simulink model "dip_student_sim_simulink_r2017b"  (R2017b)
settings: Solver=ode45  StartTime=0.0  StopTime=10  FixedStep=0.01  MaxStep=0.05  RelTol=1e-3  EnableMultiTasking=on
values from neighbouring files (symbols this model uses):
  x0 = [xR; 0; phi1R; 0; phi2R; 0]    [dip_student_sim_ini.m]
settings Model: Creator=ut  LastModifiedBy=15043
settings DataIOCC: LimitDataPoints=on  SaveFormat=Array  SignalLoggingSaveFormat=ModelDataLogs
settings OptimizationCC: ExpressionDepthLimit=2147483647  InitFltsAndDblsToZero=on  LifeSpan=inf
settings DebuggingCC: SaveWithParameterizedLinksMsg=none  UnderspecifiedInitializationDetection=Classic  MergeDetectMultiDrivingBlocksExec=none  SignalResolutionControl=TryResolveAllWithWarning  SolverPrmCheckMsg=warning  MultiTaskDSMMsg=warning  MultiTaskCondExecSysMsg=none  FcnCallInpInsideContextMsg=warning  StateNameClashWarn=warning  SFUnexpectedBacktrackingDiag=warning  SFNoUnconditionalDefaultTransitionDiag=warning  SFExecutionAtInitializationDiag=none
settings HardwareCC: ProdBitPerPointer=32  ProdBitPerSizeT=32  ProdBitPerPtrDiffT=32  ProdLargestAtomicFloat=None  ProdIntDivRoundTo=Undefined  ProdEndianess=Unspecified  ProdWordSize=32  ProdHWDeviceType=32-bit Generic
settings ModelReferenceCC: PropagateSignalLabelsOutOfModel=off
settings CodeAppCC: StateflowObjectComments=on
settings GRTTargetCC: TargetFcnLib=ansi_tfl_tmw.mat  TargetLangStandard=C89/C90 (ANSI)  CombineOutputUpdateFcns=off  GRTInterface=on
settings ConfigComp: CovMetricSettings=dw  CovSaveCumulativeToWorkspaceVar=on  CovSaveSingleToWorkspaceVar=on  CovExternalEMLEnable=off

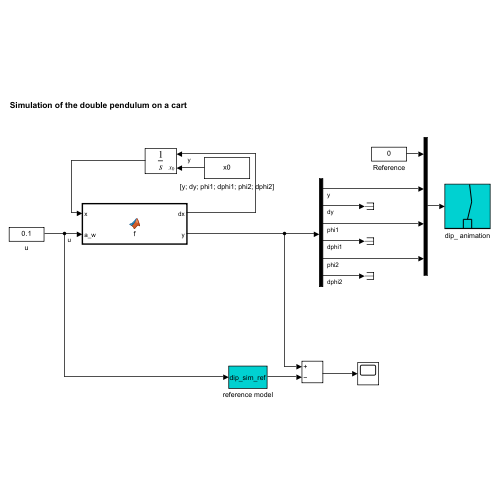
[thumbnail: Simulink's stored preview of the top-level diagram]
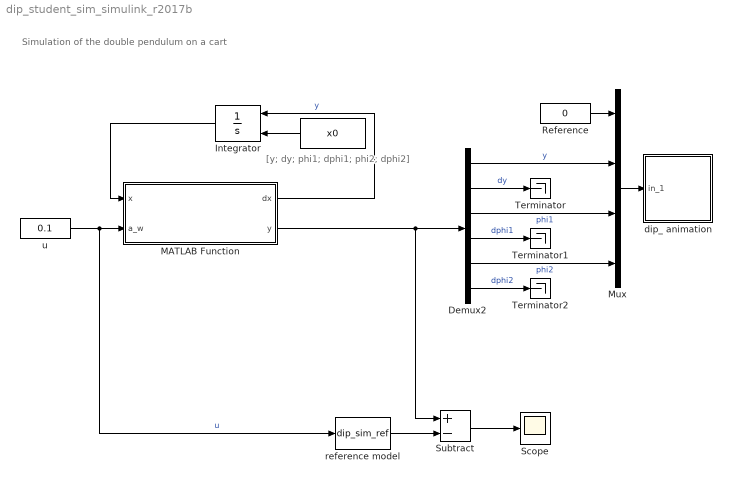
== system dip_student_sim_simulink_r2017b ==
  note: Simulation of the double pendulum on a cart
  note: [y; dy; phi1; dphi1; phi2; dphi2]
  " " : Constant  Value=x0
  Demux2 : Demux  Outputs=6
  Integrator : Integrator  InitialConditionSource=external  InitialCondition=[0;0;0;0;0;0]
  MATLAB Function : MATLAB Function  TreatAsAtomicUnit=on
  Mux : Mux
  Reference : Constant  Value=0
  Scope : Scope
  Subtract : Sum  Inputs=+-
  Terminator : Terminator
  Terminator1 : Terminator
  Terminator2 : Terminator
  dip_ animation : Subsystem  mask(Double Inverted Pendulum Plot){RefBlock=Reference}
      mask prompts: RefBlock "DC reference signal block name:"
      mask help: Double Inverted Pendulum Plot
      mask Help: Double Inverted Pendulum animation function using Handle graphics and S-function.
      mask Display: plot([-10 10],[0 0],[-2 -2 2 2],[0 1 1 0],[0 2],[1 3],[2 1],[3 5])
  reference model : M-S-Function  FunctionName=dip_sim_ref  Parameters=x0
  u : Constant  Value=0.1
  wires:
  Mux/1 -> dip_ animation/1(in_1)
  Reference/1 -> Mux/1
  u/1 -> reference model/1, MATLAB Function/2(a_w)  "u"
  MATLAB Function/1(dx) -> Integrator/1  "y"
  Demux2/1 -> Mux/2  "y"
  Demux2/3 -> Mux/3  "phi1"
  Demux2/5 -> Mux/4  "phi2"
  Demux2/2 -> Terminator/1  "dy"
  Demux2/4 -> Terminator1/1  "dphi1"
  Demux2/6 -> Terminator2/1  "dphi2"
  Subtract/1 -> Scope/1
  reference model/1 -> Subtract/2
  Integrator/1 -> MATLAB Function/1(x)
  MATLAB Function/2(y) -> Demux2/1, Subtract/1
  " "/1 -> Integrator/2

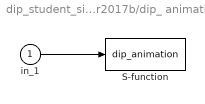
== system dip_student_sim_simulink_r2017b/dip_ animation ==
  in_1 : Inport
  S-function : S-Function  FunctionName=dip_animation  Parameters=RefBlock  SFunctionDeploymentMode=off  EnableBusSupport=off
      settings: DeleteFcn=pendan([],[],[],'DeleteBlock');
  wires:
  in_1/1 -> S-function/1

== matlab function dip_student_sim_simulink_r2017b/MATLAB Function ==
  data: x input; dx output; a_w input; y output; par parameter
function [dx, y] = f(x,a_w,par)
%YEVY
%    EXPR = YEVY(T,IN2,PARAM76,PARAM77,PARAM78,PARAM79,PARAM80,PARAM81,PARAM82,PARAM83,PARAM84,PARAM85,PARAM86,PARAM87)

%    This function was generated by the Symbolic Math Toolbox version 9.2.
%    21-Nov-2022 21:11:29

l1 = par(1);
l2 = par(2);
l_S1 = par(3);
l_S2 = par(4);
m_G1 = par(5);
m_G2 = par(6);
J_G1xx = par(7);
J_G2xx = par(8);
k_G1 = par(9);
k_G2 = par(10);
g = par(11);



%Version: 1.1
Dphi1t = x(4,:);
Dphi2t = x(6,:);
Dyt = x(2,:);
phi1 = x(3,:);
phi2 = x(5,:);
t2 = cos(phi1);
t3 = cos(phi2);
t4 = sin(phi1);
t5 = sin(phi2);
t6 = J_G1xx.*J_G2xx;
t7 = Dphi1t.^2;
t8 = Dphi2t.^2;
t9 = m_G2.^2;
t10 = l_S1.^2;
t11 = l_S2.^2;
t12 = l1.^2;
t13 = -phi2;
t14 = m_G1.*J_G2xx.*t10;
t15 = m_G2.*J_G1xx.*t11;
t16 = m_G2.*J_G2xx.*t12;
t17 = phi1+t13;
t21 = m_G1.*m_G2.*t10.*t11;
t22 = t9.*t11.*t12;
t18 = cos(t17);
t19 = sin(t17);
t20 = t18.^2;
t23 = Dphi1t.*m_G2.*k_G2.*l_S2.*l1.*t18;
t24 = Dphi2t.*m_G2.*k_G2.*l_S2.*l1.*t18;
t25 = -t24;
t26 = t20.*t22;
t27 = -t26;
t28 = t6+t14+t15+t16+t21+t22+t27;
t29 = 1.0./t28;
mt1 = [Dyt;a_w;Dphi1t;-t29.*(t23+t25+Dphi1t.*k_G1.*J_G2xx+Dphi1t.*k_G2.*J_G2xx-Dphi2t.*k_G2.*J_G2xx+t7.*t18.*t19.*t22+Dphi1t.*m_G2.*k_G1.*t11+Dphi1t.*m_G2.*k_G2.*t11-Dphi2t.*m_G2.*k_G2.*t11+a_w.*m_G1.*J_G2xx.*l_S1.*t2+a_w.*m_G2.*J_G2xx.*l1.*t2-g.*m_G1.*J_G2xx.*l_S1.*t4-g.*m_G2.*J_G2xx.*l1.*t4+a_w.*l1.*t2.*t9.*t11-g.*l1.*t4.*t9.*t11+l_S2.^3.*l1.*t8.*t9.*t19+a_w.*m_G1.*m_G2.*l_S1.*t2.*t11-g.*m_G1.*m_G2.*l_S1.*t4.*t11+m_G2.*J_G2xx.*l_S2.*l1.*t8.*t19-a_w.*l1.*t3.*t9.*t11.*t18+g.*l1.*t5.*t9.*t11.*t18);Dphi2t];
mt2 = [t29.*(t23+t25+Dphi1t.*k_G2.*J_G1xx-Dphi2t.*k_G2.*J_G1xx+t8.*t18.*t19.*t22+Dphi1t.*m_G1.*k_G2.*t10-Dphi2t.*m_G1.*k_G2.*t10+Dphi1t.*m_G2.*k_G2.*t12-Dphi2t.*m_G2.*k_G2.*t12-a_w.*m_G2.*J_G1xx.*l_S2.*t3+g.*m_G2.*J_G1xx.*l_S2.*t5-a_w.*l_S2.*t3.*t9.*t12+g.*l_S2.*t5.*t9.*t12+l_S2.*l1.^3.*t7.*t9.*t19-a_w.*m_G1.*m_G2.*l_S2.*t3.*t10+g.*m_G1.*m_G2.*l_S2.*t5.*t10+m_G2.*J_G1xx.*l_S2.*l1.*t7.*t19+a_w.*l_S2.*t2.*t9.*t12.*t18-g.*l_S2.*t4.*t9.*t12.*t18+Dphi1t.*m_G2.*k_G1.*l_S2.*l1.*t18+m_G1.*m_G2.*l_S2.*l1.*t7.*t10.*t19+a_w.*m_G1.*m_G2.*l_S1.*l_S2.*l1.*t2.*t18-g.*m_G1.*m_G2.*l_S1.*l_S2.*l1.*t4.*t18)];

dx = [mt1;mt2];
y = x;
